simulink model "sys3m_pss"  (Simulink 8.7)
settings: Solver=ode3  StartTime=0.0  StopTime=10  FixedStep=1e-2  MaxStep=1e-2  RelTol=1e-5
values from neighbouring files (symbols this model uses):
  D = 0*D    [initDyn.m]
  event = [0 1 1.10 10 ... (first row only)    [initDyn.m]
  fYred = fYGG-fYGL*inv(fYLL)*fYLG    [initDyn.m]
  KA = ExData(:,1)    [initDyn.m]
  Kpss2 = KG2*T21*T23/(T22*T24)    [initSSA.m]    (also in pss_objf.m; pss_test.m)
  Kpss3 = KG3*T31*T33/(T32*T34)    [initSSA.m]    (also in pss_objf.m; pss_test.m)
  M = 2*H/ws    [initDyn.m]
  m = 3    [initDyn.m]
  small_d = [ ... (first row only)    [initDyn.m]
  T21 = x(3)    [initSSA.m]    (also in pss_objf.m; pss_test.m)
  T22 = x(4)    [initSSA.m]    (also in pss_objf.m; pss_test.m)
  T23 = x(5)    [initSSA.m]    (also in pss_objf.m; pss_test.m)
  T24 = x(6)    [initSSA.m]    (also in pss_objf.m; pss_test.m)
  T31 = x(7)    [initSSA.m]    (also in pss_objf.m; pss_test.m)
  T32 = x(8)    [initSSA.m]    (also in pss_objf.m; pss_test.m)
  T33 = x(9)    [initSSA.m]    (also in pss_objf.m; pss_test.m)
  T34 = x(10)    [initSSA.m]    (also in pss_objf.m; pss_test.m)
  TA = ExData(:,2)    [initDyn.m]
  Tpd0 = GenData(:,6)    [initDyn.m]
  Tpq0 = GenData(:,7)    [initDyn.m]
  Tw = 10    [initSSA.m]    (also in pss_objf.m; pss_test.m)
  ws = 377    [initDyn.m]
  XXdpd = [Xd-Xpd]    [initDyn.m]
  XXpdq = [Xpq-Xpd]    [initDyn.m]
  XXqpq = [Xq-Xpq]    [initDyn.m]
  Yred = YGG-YGL*inv(YLL)*YLG    [initDyn.m]
  Zdq = [Rsm -Xpqm;Xpdm Rsm]    [initDyn.m]
undefined symbols (not defined in the file or in its folder): delta0, Efd0, Epd0, Epq0, Vref1
libraries: powerlib_extras x2
settings Model: Creator=hbeiran  LastModifiedBy=EBUKA
settings SolverCC: AlgebraicLoopSolver=LineSearch
settings DataIOCC: LimitDataPoints=off  SignalLoggingSaveFormat=ModelDataLogs
settings OptimizationCC: ExpressionDepthLimit=2147483647
settings DebuggingCC: AlgebraicLoopMsg=none  SolverPrmCheckMsg=warning  FcnCallInpInsideContextMsg=UseLocalSettings  StateNameClashWarn=warning  StrictBusMsg=Warning
settings SFSimCC: SimParseCustomCode=off
settings GRTTargetCC: CombineOutputUpdateFcns=off  GRTInterface=on

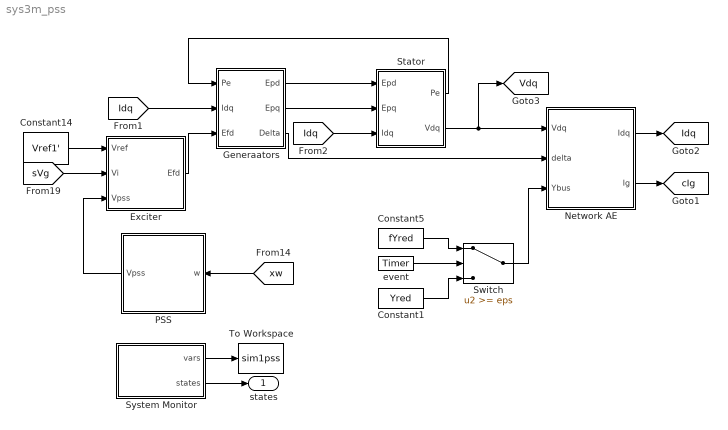
== system sys3m_pss ==
  Constant1 : Constant  Value=Yred  VectorParams1D=off
  Constant14 : Constant  Value=Vref1'  VectorParams1D=off
  Constant5 : Constant  Value=fYred  VectorParams1D=off
  Exciter : Subsystem
  Generaators : Subsystem
  Network AE : MATLAB Function  TreatAsAtomicUnit=on
  PSS : Subsystem
  Stator : Subsystem
  Switch : Switch  Threshold=eps
  System Monitor : Subsystem
  To Workspace : ToWorkspace  VariableName=sim1pss  SaveFormat=Structure With Time  SampleTime=-1
  event : powerlib_extras/Control  Blocks/Timer  t=event(1,:)  e=event(2,:)
  states : Outport
  tag scope: Idq=global, Vdq=global, cIg=global
  wires:
  Exciter/1(Efd) -> Generaators/3(Efd)
  Constant14/1 -> Exciter/1(Vref)
  [Idq] -> Generaators/2(Idq)
  Network AE/1(Idq) -> [Idq]
  event/1 -> Switch/2
  Constant5/1 -> Switch/1
  Constant1/1 -> Switch/3
  Switch/1 -> Network AE/3(Ybus)
  System Monitor/1(vars) -> To Workspace/1
  System Monitor/2(states) -> states/1
  Generaators/3(Delta) -> Network AE/2(delta)
  Network AE/2(Ig) -> [cIg]
  Stator/2(Vdq) -> Network AE/1(Vdq), [Vdq]
  [Idq] -> Stator/3(Idq)
  Generaators/1(Epd) -> Stator/1(Epd)
  Generaators/2(Epq) -> Stator/2(Epq)
  Stator/1(Pe) -> Generaators/1(Pe)
  [sVg] -> Exciter/2(Vi)
  PSS/1(Vpss) -> Exciter/3(Vpss)
  [xw] -> PSS/1(w)

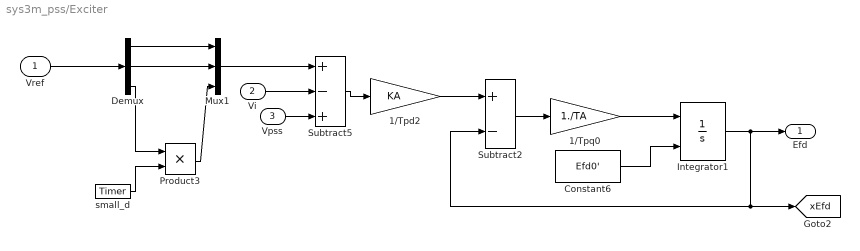
== system sys3m_pss/Exciter ==
  Vref : Inport
  Vi : Inport  Port=2
  Vpss : Inport  Port=3
  1/Tpd2 : Gain  Gain=KA
  1/Tpq0 : Gain  Gain=1./TA
  Constant6 : Constant  Value=Efd0'  VectorParams1D=off
  Demux : Demux  Outputs=3
  Integrator1 : Integrator  InitialConditionSource=external
  Mux1 : Mux  Inputs=3
  Product3 : Product  RndMeth=Zero
  Subtract2 : Sum  Inputs=+-
  Subtract5 : Sum  Inputs=+-+
  small_d : powerlib_extras/Control  Blocks/Timer  t=small_d(1,:)  e=small_d(2,:)
  Efd : Outport
  tag scope: xEfd=global
  wires:
  Constant6/1 -> Integrator1/2
  Subtract2/1 -> 1/Tpq0/1
  1/Tpq0/1 -> Integrator1/1
  Integrator1/1 -> Efd/1, Subtract2/2, [xEfd]
  Vi/1 -> Subtract5/2
  Subtract5/1 -> 1/Tpd2/1
  1/Tpd2/1 -> Subtract2/1
  Demux/1 -> Mux1/1
  Demux/2 -> Mux1/2
  Demux/3 -> Product3/1
  Product3/1 -> Mux1/3
  small_d/1 -> Product3/2
  Mux1/1 -> Subtract5/1
  Vref/1 -> Demux/1
  Vpss/1 -> Subtract5/3

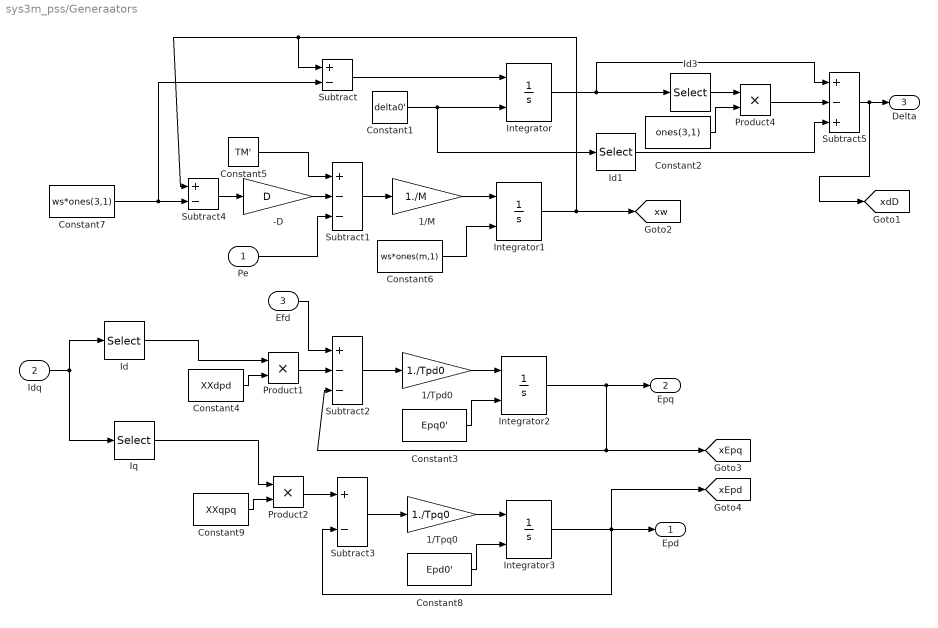
== system sys3m_pss/Generaators ==
  Pe : Inport
  Idq : Inport  Port=2
  Efd : Inport  Port=3
  -D : Gain  Gain=D
  1/M : Gain  Gain=1./M
  1/Tpd0 : Gain  Gain=1./Tpd0
  1/Tpq0 : Gain  Gain=1./Tpq0
  Constant1 : Constant  Value=delta0'  VectorParams1D=off
  Constant2 : Constant  Value=ones(3,1)  VectorParams1D=off
  Constant3 : Constant  Value=Epq0'  VectorParams1D=off
  Constant4 : Constant  Value=XXdpd  VectorParams1D=off
  Constant5 : Constant  Value=TM'  VectorParams1D=off
  Constant6 : Constant  Value=ws*ones(m,1)  VectorParams1D=off
  Constant7 : Constant  Value=ws*ones(3,1)  VectorParams1D=off
  Constant8 : Constant  Value=Epd0'  VectorParams1D=off
  Constant9 : Constant  Value=XXqpq  VectorParams1D=off
  Id : Selector  InputPortWidth=6  IndexOptions=Index vector (dialog)  Indices=[1:3]  OutputSizes=1
  Id1 : Selector  InputPortWidth=3  IndexOptions=Index vector (dialog)  Indices=[1]  OutputSizes=1
  Id3 : Selector  InputPortWidth=3  IndexOptions=Index vector (dialog)  Indices=[1]  OutputSizes=1
  Integrator{,1..3} (4 alike) : Integrator  InitialConditionSource=external
  Iq : Selector  InputPortWidth=6  IndexOptions=Index vector (dialog)  Indices=[4:6]  OutputSizes=1
  Product1 : Product  RndMeth=Zero
  Product2 : Product  RndMeth=Zero
  Product4 : Product  RndMeth=Zero
  Subtract : Sum  Inputs=+-
  Subtract1 : Sum  Inputs=+--
  Subtract2 : Sum  Inputs=+--
  Subtract3 : Sum  Inputs=+-
  Subtract4 : Sum  Inputs=+-
  Subtract5 : Sum  Inputs=+-+
  Epd : Outport
  Epq : Outport  Port=2
  Delta : Outport  Port=3
  tag scope: xEpd=global, xEpq=global, xdD=global, xw=global
  wires:
  Subtract/1 -> Integrator/1
  Constant5/1 -> Subtract1/1
  Subtract1/1 -> 1/M/1
  1/M/1 -> Integrator1/1
  Constant6/1 -> Integrator1/2
  -D/1 -> Subtract1/2
  Constant3/1 -> Integrator2/2
  Subtract2/1 -> 1/Tpd0/1
  Integrator2/1 -> Epq/1, Subtract2/3, [xEpq]
  Product1/1 -> Subtract2/2
  Constant4/1 -> Product1/2
  1/Tpd0/1 -> Integrator2/1
  Constant8/1 -> Integrator3/2
  Subtract3/1 -> 1/Tpq0/1
  Integrator3/1 -> Subtract3/2, Epd/1, [xEpd]
  Constant9/1 -> Product2/2
  1/Tpq0/1 -> Integrator3/1
  Product2/1 -> Subtract3/1
  Efd/1 -> Subtract2/1
  Integrator1/1 -> [xw], Subtract/1, Subtract4/1
  Id/1 -> Product1/1
  Idq/1 -> Id/1, Iq/1
  Iq/1 -> Product2/1
  Pe/1 -> Subtract1/3
  Subtract4/1 -> -D/1
  Constant7/1 -> Subtract4/2, Subtract/2
  Subtract5/1 -> Delta/1, [xdD]
  Constant1/1 -> Integrator/2, Id1/1
  Integrator/1 -> Subtract5/1, Id3/1
  Id3/1 -> Product4/1
  Constant2/1 -> Product4/2
  Product4/1 -> Subtract5/2
  Id1/1 -> Subtract5/3

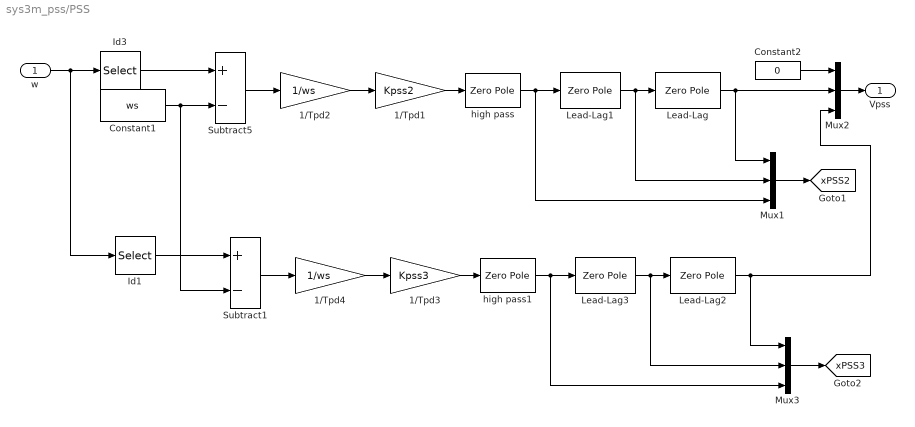
== system sys3m_pss/PSS ==
  w : Inport
  1/Tpd1 : Gain  Gain=Kpss2
  1/Tpd2 : Gain  Gain=1/ws
  1/Tpd3 : Gain  Gain=Kpss3
  1/Tpd4 : Gain  Gain=1/ws
  Constant1 : Constant  Value=ws  VectorParams1D=off
  Constant2 : Constant  Value=0  VectorParams1D=off
  Id1 : Selector  InputPortWidth=3  IndexOptions=Index vector (dialog)  Indices=[3]  OutputSizes=1
  Id3 : Selector  InputPortWidth=3  IndexOptions=Index vector (dialog)  Indices=[2]  OutputSizes=1
  Lead-Lag : ZeroPole  Zeros=[-1/T23]  Poles=[-1/T24]
  Lead-Lag1 : ZeroPole  Zeros=[-1/T21]  Poles=[-1/T22]
  Lead-Lag2 : ZeroPole  Zeros=[-1/T33]  Poles=[-1/T34]
  Lead-Lag3 : ZeroPole  Zeros=[-1/T31]  Poles=[-1/T32]
  Mux1 : Mux  Inputs=3
  Mux2 : Mux  Inputs=3
  Mux3 : Mux  Inputs=3
  Subtract1 : Sum  Inputs=+-
  Subtract5 : Sum  Inputs=+-
  high pass : ZeroPole  Zeros=[0]  Poles=[-1/Tw]
  high pass1 : ZeroPole  Zeros=[0]  Poles=[-1/Tw]
  Vpss : Outport
  tag scope: xPSS2=global, xPSS3=global
  wires:
  Subtract5/1 -> 1/Tpd2/1
  1/Tpd1/1 -> high pass/1
  Lead-Lag/1 -> Mux1/1, Mux2/2
  w/1 -> Id3/1, Id1/1
  high pass/1 -> Lead-Lag1/1, Mux1/3
  Lead-Lag1/1 -> Lead-Lag/1, Mux1/2
  Mux1/1 -> [xPSS2]
  1/Tpd2/1 -> 1/Tpd1/1
  Mux2/1 -> Vpss/1
  Constant2/1 -> Mux2/1
  Id3/1 -> Subtract5/1
  Constant1/1 -> Subtract5/2, Subtract1/2
  Subtract1/1 -> 1/Tpd4/1
  1/Tpd3/1 -> high pass1/1
  Lead-Lag2/1 -> Mux3/1, Mux2/3
  high pass1/1 -> Mux3/3, Lead-Lag3/1
  Lead-Lag3/1 -> Mux3/2, Lead-Lag2/1
  Mux3/1 -> [xPSS3]
  1/Tpd4/1 -> 1/Tpd3/1
  Id1/1 -> Subtract1/1

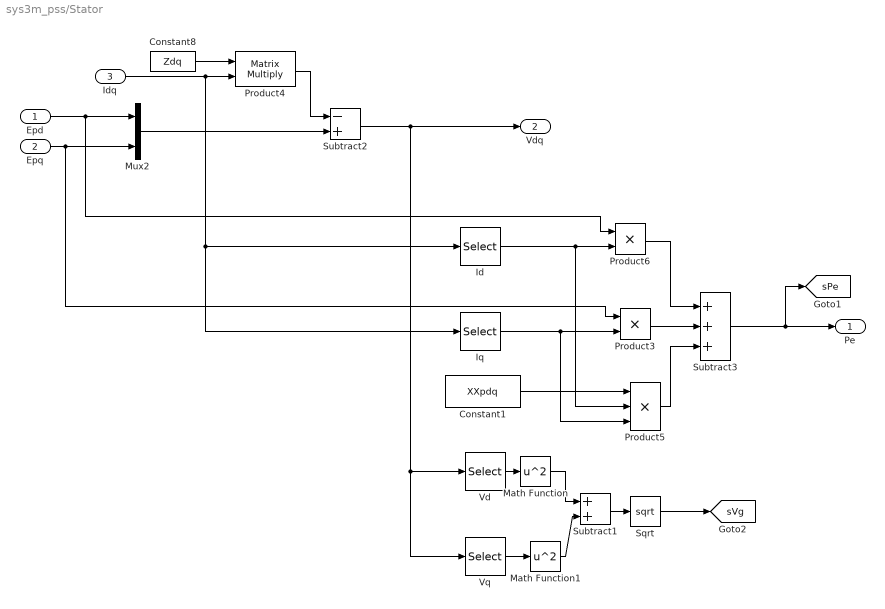
== system sys3m_pss/Stator ==
  Epd : Inport
  Epq : Inport  Port=2
  Idq : Inport  Port=3
  Constant1 : Constant  Value=XXpdq  VectorParams1D=off
  Constant8 : Constant  Value=Zdq  VectorParams1D=off
  Id : Selector  InputPortWidth=6  IndexOptions=Index vector (dialog)  Indices=[1:3]  OutputSizes=1
  Iq : Selector  InputPortWidth=6  IndexOptions=Index vector (dialog)  Indices=[4:6]  OutputSizes=1
  Math Function : Math  Operator=square  SaturateOnIntegerOverflow=on
  Math Function1 : Math  Operator=square  SaturateOnIntegerOverflow=on
  Mux2 : Mux  Inputs=2
  Product3 : Product  RndMeth=Zero
  Product4 : Product  Multiplication=Matrix(*)  RndMeth=Zero
  Product5 : Product  Inputs=3  RndMeth=Zero
  Product6 : Product  RndMeth=Zero
  Sqrt : Sqrt  SaturateOnIntegerOverflow=on
  Subtract1 : Sum
  Subtract2 : Sum  Inputs=-+
  Subtract3 : Sum  Inputs=+++
  Vd : Selector  InputPortWidth=6  IndexOptions=Index vector (dialog)  Indices=[1:3]  OutputSizes=1
  Vq : Selector  InputPortWidth=6  IndexOptions=Index vector (dialog)  Indices=[4:6]  OutputSizes=1
  Pe : Outport
  Vdq : Outport  Port=2
  tag scope: sPe=global, sVg=global
  wires:
  Constant8/1 -> Product4/1
  Epd/1 -> Mux2/1, Product6/1
  Epq/1 -> Product3/1, Mux2/2
  Iq/1 -> Product5/3, Product3/2
  Product6/1 -> Subtract3/1
  Product3/1 -> Subtract3/2
  Product5/1 -> Subtract3/3
  Constant1/1 -> Product5/1
  Subtract3/1 -> Pe/1, [sPe]
  Id/1 -> Product6/2, Product5/2
  Vd/1 -> Math Function/1
  Vq/1 -> Math Function1/1
  Math Function/1 -> Subtract1/1
  Math Function1/1 -> Subtract1/2
  Subtract1/1 -> Sqrt/1
  Sqrt/1 -> [sVg]
  Mux2/1 -> Subtract2/2
  Idq/1 -> Product4/2, Id/1, Iq/1
  Product4/1 -> Subtract2/1
  Subtract2/1 -> Vdq/1, Vq/1, Vd/1

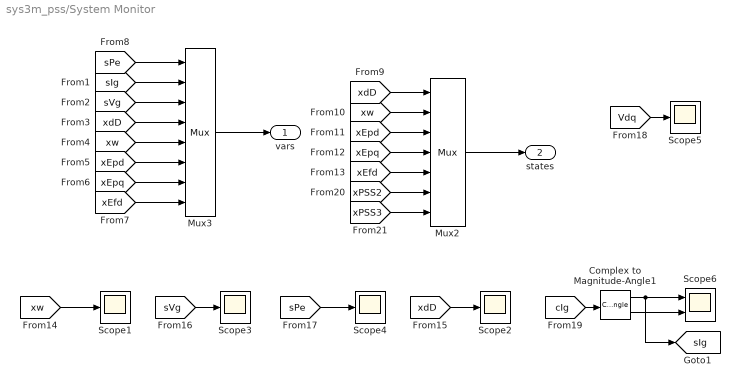
== system sys3m_pss/System Monitor ==
  Complex to Magnitude-Angle1 : ComplexToMagnitudeAngle
  Mux2 : Mux  Inputs=7
  Mux3 : Mux  Inputs=8
  Scope{1..5} (5 alike) : Scope
  Scope6 : Scope  NumInputPorts=2
  vars : Outport
  states : Outport  Port=2
  tag scope: sIg=global
  wires:
  Mux3/1 -> vars/1
  [sPe] -> Mux3/1
  [sIg] -> Mux3/2
  [sVg] -> Mux3/3
  [xdD] -> Mux3/4
  [xw] -> Mux3/5
  [xEpd] -> Mux3/6
  [xEpq] -> Mux3/7
  [xEfd] -> Mux3/8
  [xw] -> Mux2/2
  [xEpd] -> Mux2/3
  [xEpq] -> Mux2/4
  [xEfd] -> Mux2/5
  [xdD] -> Mux2/1
  Mux2/1 -> states/1
  [xw] -> Scope1/1
  [xdD] -> Scope2/1
  [sVg] -> Scope3/1
  [sPe] -> Scope4/1
  Complex to Magnitude-Angle1/1 -> Scope6/1, [sIg]
  Complex to Magnitude-Angle1/2 -> Scope6/2
  [cIg] -> Complex to Magnitude-Angle1/1
  [Vdq] -> Scope5/1
  [xPSS2] -> Mux2/6
  [xPSS3] -> Mux2/7

== matlab function Network AE ==
  data: Vdq input double; Idq output double; delta input double; Ig output double; Ybus input double
function [Idq, Ig] = fcn(Vdq,delta,Ybus)
%#codegen
% global_var

% Idq

Tm = diag(exp(1j*(delta-pi/2)));
iTm = diag(exp(-1j*(delta-pi/2)));
% iTm = inv(Tm);
% Tm=eye(3);
Vg = Tm*(Vdq(1:3,1)+1j*Vdq(4:6,1));
% VLoad=VL(4:9,1);
% Vbus=[Vg;VLoad];


I = Ybus*Vg;
Ig=I(1:3,1);
Id=real(iTm*Ig);
Iq=imag(iTm*Ig);

Idq=[Id;Iq];
